simulink model "Quarter_car_model"  (R2024b)
settings: Solver=FixedStepAuto  StartTime=0.0  StopTime=100  FixedStep=0.01  RelTol=1e-3
values from neighbouring files (symbols this model uses):
  cdamper = 1500    [Quarter_car_model_parameters.m]
  F0 = 3924    [Quarter_car_model_parameters.m]
  g = 9.81    [Quarter_car_model_parameters.m]
  kspring = 35500    [Quarter_car_model_parameters.m]
  ktyre = 300000    [Quarter_car_model_parameters.m]
  ms = 400    [Quarter_car_model_parameters.m]
  mus = 30    [Quarter_car_model_parameters.m]
  z0tyre = (ms+mus)*g/ktyre    (= 0.014061)    [Quarter_car_model_parameters.m]
libraries: simulink x1
settings Model: Creator=jayku  LastModifiedBy=jayku

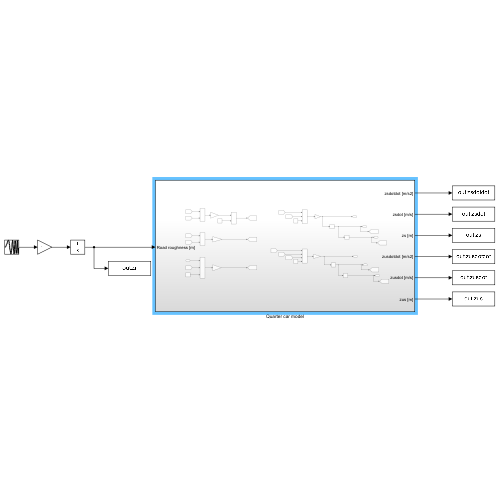
[thumbnail: Simulink's stored preview of the top-level diagram]
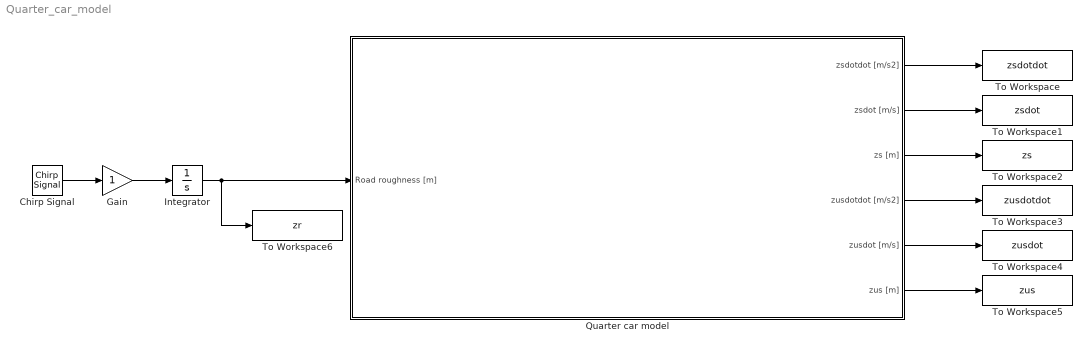
== system Quarter_car_model ==
  Chirp Signal : simulink/Sources/Chirp Signal  f1=0.1  T=100  f2=50
  Gain : Gain
  Integrator : Integrator
  Quarter car model : Subsystem
  To Workspace : ToWorkspace  VariableName=zsdotdot  SaveFormat=Timeseries  SampleTime=-1
  To Workspace1 : ToWorkspace  VariableName=zsdot  SaveFormat=Timeseries  SampleTime=-1
  To Workspace2 : ToWorkspace  VariableName=zs  SaveFormat=Timeseries  SampleTime=-1
  To Workspace3 : ToWorkspace  VariableName=zusdotdot  SaveFormat=Timeseries  SampleTime=-1
  To Workspace4 : ToWorkspace  VariableName=zusdot  SaveFormat=Timeseries  SampleTime=-1
  To Workspace5 : ToWorkspace  VariableName=zus  SaveFormat=Timeseries  SampleTime=-1
  To Workspace6 : ToWorkspace  VariableName=zr  SaveFormat=Timeseries  SampleTime=-1
  wires:
  Quarter car model/1(zsdotdot [m/s2]) -> To Workspace/1
  Quarter car model/2(zsdot [m/s]) -> To Workspace1/1
  Quarter car model/3(zs [m]) -> To Workspace2/1
  Quarter car model/4(zusdotdot [m/s2]) -> To Workspace3/1
  Quarter car model/5(zusdot [m/s]) -> To Workspace4/1
  Quarter car model/6(zus [m]) -> To Workspace5/1
  Integrator/1 -> Quarter car model/1(Road roughness [m]), To Workspace6/1
  Gain/1 -> Integrator/1
  Chirp Signal/1 -> Gain/1

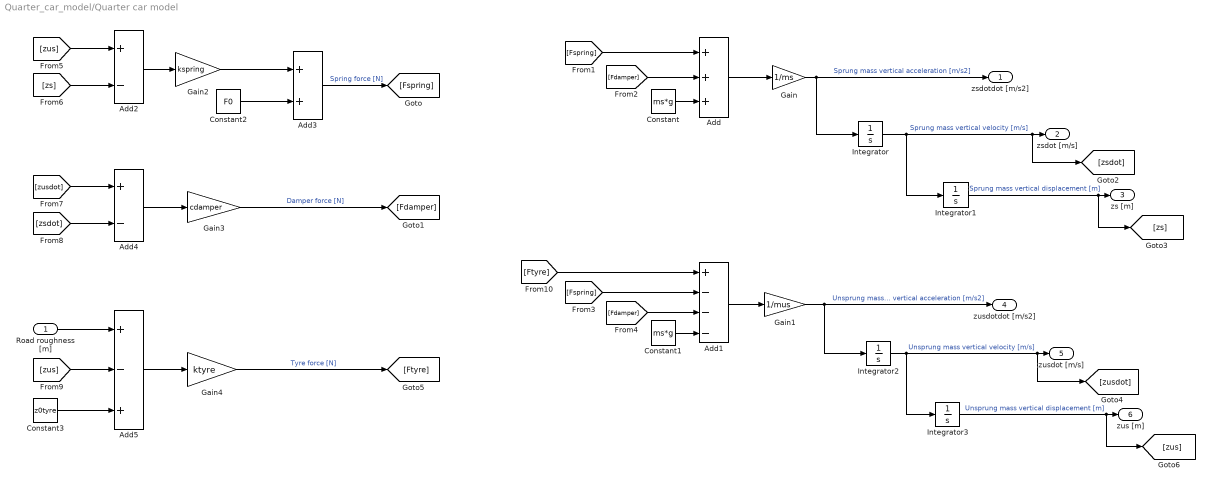
== system Quarter_car_model/Quarter car model ==
  Road roughness [m] : Inport
  Add : Sum  Inputs=+++
  Add1 : Sum  Inputs=+---
  Add2 : Sum  Inputs=+-
  Add3 : Sum
  Add4 : Sum  Inputs=+-
  Add5 : Sum  Inputs=+-+
  Constant : Constant  Value=ms*g
  Constant1 : Constant  Value=ms*g
  Constant2 : Constant  Value=F0
  Constant3 : Constant  Value=z0tyre
  Gain : Gain  Gain=1/ms
  Gain1 : Gain  Gain=1/mus
  Gain2 : Gain  Gain=kspring
  Gain3 : Gain  Gain=cdamper
  Gain4 : Gain  Gain=ktyre
  Integrator{,1..3} (4 alike) : Integrator
  zsdotdot [m/s2] : Outport
  zsdot [m/s] : Outport  Port=2
  zs [m] : Outport  Port=3
  zusdotdot [m/s2] : Outport  Port=4
  zusdot [m/s] : Outport  Port=5
  zus [m] : Outport  Port=6
  wires:
  Add/1 -> Gain/1
  Gain/1 -> Integrator/1, zsdotdot [m/s2]/1  "Sprung mass vertical acceleration [m/s2]"
  Integrator/1 -> [zsdot], zsdot [m/s]/1, Integrator1/1  "Sprung mass vertical velocity [m/s]"
  Integrator1/1 -> [zs], zs [m]/1  "Sprung mass vertical displacement [m]"
  Constant/1 -> Add/3
  [Fdamper] -> Add/2
  [Fspring] -> Add/1
  Gain1/1 -> zusdotdot [m/s2]/1, Integrator2/1  "Unsprung mass vertical acceleration [m/s2]"
  Add1/1 -> Gain1/1
  Integrator2/1 -> [zusdot], zusdot [m/s]/1, Integrator3/1  "Unsprung mass vertical velocity [m/s]"
  Integrator3/1 -> [zus], zus [m]/1  "Unsprung mass vertical displacement [m]"
  Constant1/1 -> Add1/4
  [Fdamper] -> Add1/3
  [Fspring] -> Add1/2
  Add2/1 -> Gain2/1
  [zs] -> Add2/2
  [zus] -> Add2/1
  Gain2/1 -> Add3/1
  Constant2/1 -> Add3/2
  Add3/1 -> [Fspring]  "Spring force [N]"
  [zusdot] -> Add4/1
  [zsdot] -> Add4/2
  Add4/1 -> Gain3/1
  Gain3/1 -> [Fdamper]  "Damper force [N]"
  Road roughness [m]/1 -> Add5/1
  Constant3/1 -> Add5/3
  [zus] -> Add5/2
  Add5/1 -> Gain4/1
  Gain4/1 -> [Ftyre]  "Tyre force [N]"
  [Ftyre] -> Add1/1
